simulink model "ep_5_4"  (R2023b)
settings: Solver=VariableStepAuto  StartTime=0.0  StopTime=10.0  RelTol=1e-3
libraries: ep5_lib x1
settings Model: Creator=86186  LastModifiedBy=86186

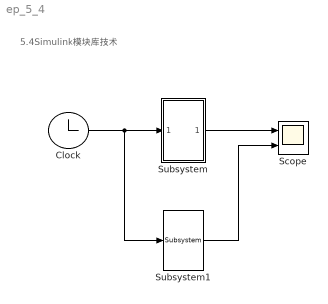
== system ep_5_4 ==
  note: 5.4Simulink模块库技术
  Clock : Clock
  Scope : Scope  NumInputPorts=2
  Subsystem : Subsystem  AncestorBlock=ep5_lib/Subsystem  mask{a=3, b=4}
      mask init:
      | t = 0:0.1:2;
      | y = 3*t +4;
      mask DialogControl ParameterGroupVar Prompt: 参数
      mask Display:
      | plot(t,y);
      | port_label('input', 1, 'in');
      | port_label('output', 1, 'out');
  Subsystem1 : ep5_lib/Subsystem  a=3  b=4
  wires:
  Subsystem/1(Out1) -> Scope/1
  Clock/1 -> Subsystem1/1, Subsystem/1(In1)
  Subsystem1/1 -> Scope/2

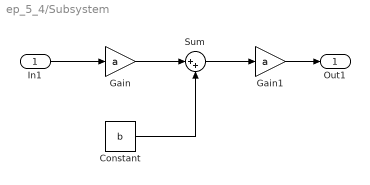
== system ep_5_4/Subsystem ==
  In1 : Inport
  Constant : Constant  Value=b
  Gain : Gain  Gain=a
  Gain1 : Gain  Gain=a
  Sum : Sum  Inputs=|++
  Out1 : Outport
  wires:
  Sum/1 -> Gain1/1
  In1/1 -> Gain/1
  Gain/1 -> Sum/1
  Constant/1 -> Sum/2
  Gain1/1 -> Out1/1
